simulink model "simulation"  (R2014a)
settings: Solver=ode45  StartTime=0.0  StopTime=25  RelTol=1e-3
values from neighbouring files (symbols this model uses):
  C = C(1:2,:)    [timeInvLQG.m]
  g = 9.82    [est_JB.m]    (also in generatePaths.m)
  Gamma = Gamma(:,1)    [timeInvLQG.m]
  h = s.h    [generatePaths.m]    (also in throwPath.mat = 0.01; timeInvLQG.m = 0.01)
  JB = JN    [BallAndBeam.m]    (also in est_JB.m = mean(JB_samples))
  K = K(:,1:2)    [timeInvLQG.m]
  kB = kB_ku * ku    (= -0.946243109081)    [est_JB.m]
  ku = m_weigh*g*x_weigh / u_weigh    (= 0.309657333333)    [est_JB.m]
  L = L(1,:)    [timeInvLQG.m]
  m = 0.1    [timeInvLQG.m]
  Phi = discsys.a    [timeInvLQG.m]
  u0 = -(-m*g*x1*cos(0)+kB*0)/ku    [timeInvLQG.m]
  x0 = [x1; 0; 0; 0; m; 0]    [timeInvLQG.m]
  x1 = 0.3    [timeInvLQG.m]
  x10 = 0.1    [timeInvLQG.m]
  x20 = 0    [timeInvLQG.m]
  x30 = 0    [timeInvLQG.m]
  x40 = 0    [timeInvLQG.m]
settings Model: Creator=Mattias  LastModifiedBy=Mattias

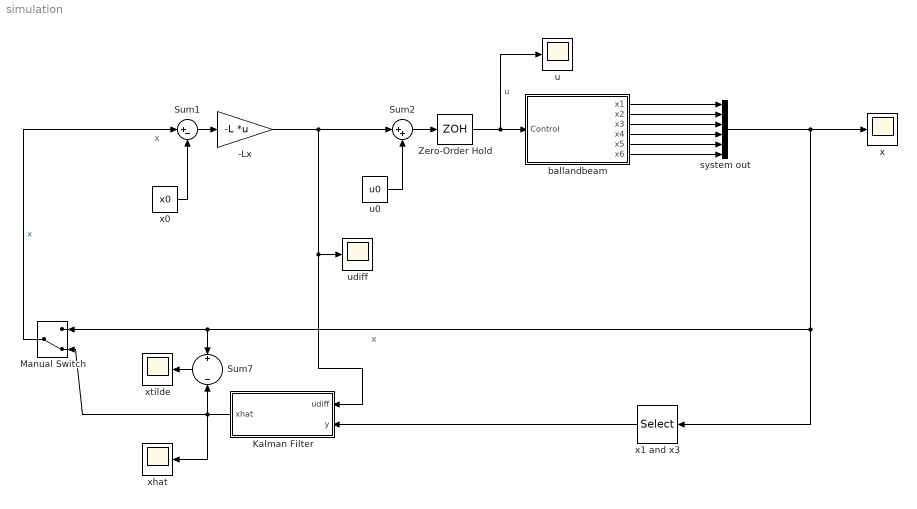
== system simulation ==
  note: x
  note: x
  -Lx : Gain  Gain=-L  Multiplication=Matrix(K*u) (u vector)
  Kalman Filter : Subsystem
  Manual Switch : ManualSwitch  CurrentSetting=0
  Sum1 : Sum  Inputs=|+-
  Sum2 : Sum  Inputs=|++
  Sum7 : Sum  Inputs=+||-
  Zero-Order Hold : ZeroOrderHold  SampleTime=h
  ballandbeam : Subsystem
  system out : Concatenate  NumInputs=6
  u : Scope
      settings: ShowLegends=on
  u0 : Constant  Value=u0
  udiff : Scope
      settings: ShowLegends=on  SaveName=ScopeData6
  x : Scope
      settings: ShowLegends=on
  x0 : Constant  Value=x0
  x1 and x3 : Selector  InputPortWidth=6  Indices=[1 3]
  xhat : Scope
      settings: ShowLegends=on  SaveName=ScopeData2
  xtilde : Scope
      settings: ShowLegends=on  SaveName=ScopeData3
  wires:
  Zero-Order Hold/1 -> u/1, ballandbeam/1(Control)  "u"
  Sum1/1 -> -Lx/1
  x0/1 -> Sum1/2
  -Lx/1 -> Sum2/1, Kalman Filter/1(udiff), udiff/1
  Sum2/1 -> Zero-Order Hold/1
  u0/1 -> Sum2/2
  Manual Switch/1 -> Sum1/1  "x"
  Kalman Filter/1(xhat) -> xhat/1, Manual Switch/2, Sum7/2
  system out/1 -> Manual Switch/1, Sum7/1, x1 and x3/1, x/1
  Sum7/1 -> xtilde/1
  x1 and x3/1 -> Kalman Filter/2(y)
  ballandbeam/1(x1) -> system out/1
  ballandbeam/3(x3) -> system out/3
  ballandbeam/4(x4) -> system out/4
  ballandbeam/2(x2) -> system out/2
  ballandbeam/5(x5) -> system out/5
  ballandbeam/6(x6) -> system out/6

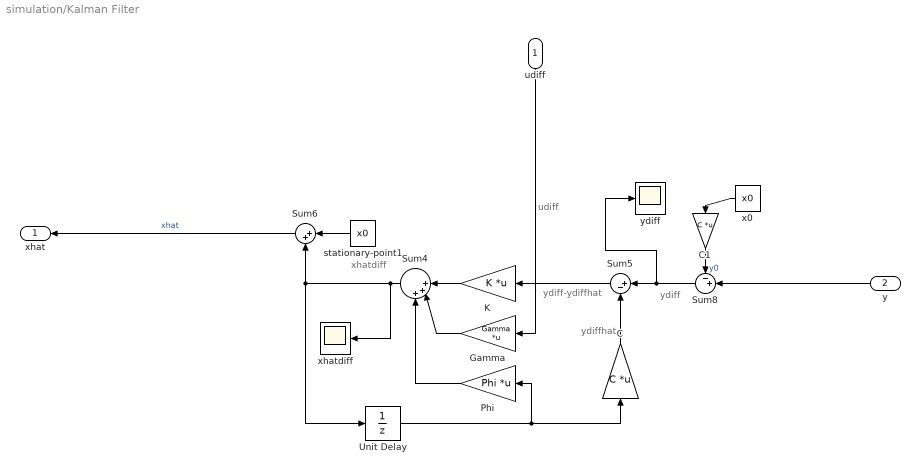
== system simulation/Kalman Filter ==
  note: ydiff
  note: ydiffhat
  note: ydiff-ydiffhat
  note: udiff
  note: xhatdiff
  udiff : Inport
  y : Inport  Port=2
  C : Gain  Gain=C  Multiplication=Matrix(K*u) (u vector)
  C1 : Gain  Gain=C  Multiplication=Matrix(K*u) (u vector)
  Gamma : Gain  Gain=Gamma  Multiplication=Matrix(K*u) (u vector)
  K : Gain  Gain=K  Multiplication=Matrix(K*u) (u vector)
  Phi : Gain  Gain=Phi  Multiplication=Matrix(K*u) (u vector)
  Sum4 : Sum  Inputs=||+++
  Sum5 : Sum  Inputs=|+-
  Sum6 : Sum  Inputs=|++
  Sum8 : Sum  Inputs=-+|
  Unit Delay : UnitDelay  SampleTime=h
  stationary-point1 : Constant  Value=x0
  x0 : Constant  Value=x0
  xhatdiff : Scope
      settings: ShowLegends=on  SaveName=ScopeData8
  ydiff : Scope
      settings: ShowLegends=on  SaveName=ScopeData10
  xhat : Outport
  wires:
  udiff/1 -> Gamma/1
  Phi/1 -> Sum4/3
  Gamma/1 -> Sum4/2
  K/1 -> Sum4/1
  C/1 -> Sum5/2
  Sum5/1 -> K/1
  Sum4/1 -> xhatdiff/1, Unit Delay/1, Sum6/2
  Unit Delay/1 -> C/1, Phi/1
  stationary-point1/1 -> Sum6/1
  x0/1 -> C1/1
  y/1 -> Sum8/2
  C1/1 -> Sum8/1  "y0"
  Sum8/1 -> ydiff/1, Sum5/1
  Sum6/1 -> xhat/1  "xhat"

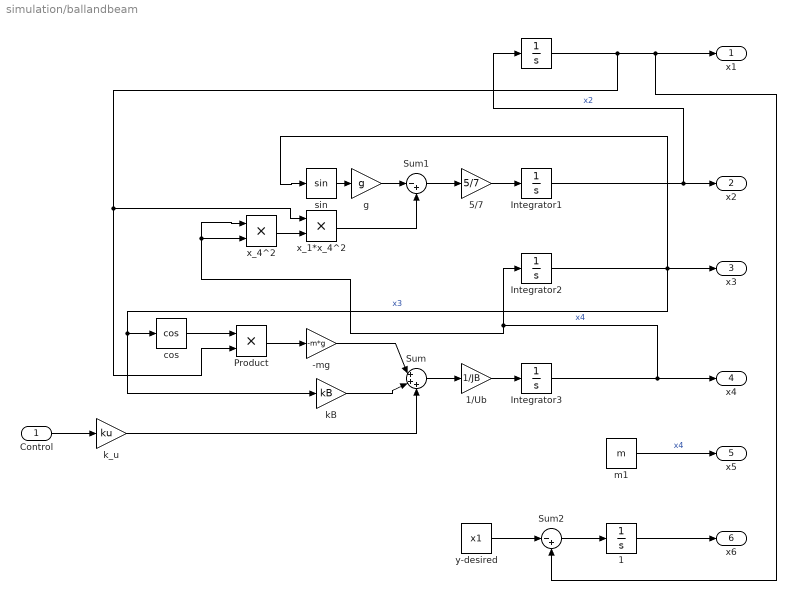
== system simulation/ballandbeam ==
  Control : Inport
  "\t" : Integrator  InitialCondition=x10
  "\t1" : Integrator
  -mg : Gain  Gain=-m*g
  1/Ub : Gain  Gain=1/JB
  5/7 : Gain  Gain=5/7
  Integrator1 : Integrator  InitialCondition=x20
  Integrator2 : Integrator  InitialCondition=x30
  Integrator3 : Integrator  InitialCondition=x40
  Product : Product
  Sum : Sum  Inputs=|+++
  Sum1 : Sum  Inputs=|-+
  Sum2 : Sum  Inputs=|-+
  cos : Trigonometry  Operator=cos
  g : Gain  Gain=g
  kB : Gain  Gain=kB
  k_u : Gain  Gain=ku
  m1 : Constant  Value=m
  sin : Trigonometry
  x_1*x_4^2 : Product
  x_4^2 : Product
  y-desired : Constant  Value=x1
  x1 : Outport
  x2 : Outport  Port=2
  x3 : Outport  Port=3
  x4 : Outport  Port=4
  x5 : Outport  Port=5
  x6 : Outport  Port=6
  wires:
  Control/1 -> k_u/1
  Product/1 -> -mg/1
  1/Ub/1 -> Integrator3/1
  cos/1 -> Product/1
  Sum/1 -> 1/Ub/1
  -mg/1 -> Sum/1
  kB/1 -> Sum/2
  k_u/1 -> Sum/3
  5/7/1 -> Integrator1/1
  Sum1/1 -> 5/7/1
  sin/1 -> g/1
  g/1 -> Sum1/1
  x_4^2/1 -> x_1*x_4^2/2
  x_1*x_4^2/1 -> Sum1/2
  "\t"/1 -> Sum2/2, x1/1, x_1*x_4^2/1, Product/2
  Integrator1/1 -> "\t"/1, x2/1  "x2"
  Integrator2/1 -> kB/1, cos/1, sin/1, x3/1  "x3"
  Integrator3/1 -> x_4^2/2, x_4^2/1, Integrator2/1, x4/1  "x4"
  m1/1 -> x5/1  "x4"
  "\t1"/1 -> x6/1
  Sum2/1 -> "\t1"/1
  y-desired/1 -> Sum2/1
